simulink model "interpolation_nD_TestGen61"  (R2017b)
settings: Solver=FixedStepDiscrete  StartTime=0.0  StopTime=10.0  RelTol=1e-3
settings Model: Creator=ktrinh  LastModifiedBy=ktrinh
settings DebuggingCC: ParameterOverflowMsg=none

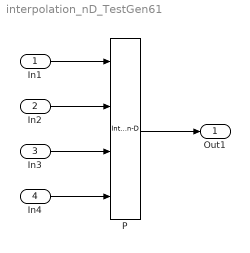
== system interpolation_nD_TestGen61 ==
  In1 : Inport  OutMax=2
  In2 : Inport  Port=2  OutMax=5
  In3 : Inport  Port=3  OutMax=3
  In4 : Inport  Port=4  OutMin=0  OutMax=2
  P : Interpolation_n-D  NumberOfTableDimensions=4  Table=reshape(repmat([4 5 6 7 8;16 19 20 21 22;10 18 23 24 25],2,2),[2,5,3,2])  InterpMethod=Nearest  ValidIndexMayReachLast=on  NumSelectionDims=4  InternalRulePriority=Speed  RndMeth=Simplest  SaturateOnIntegerOverflow=on  IntermediateResultsDataTypeStr=uint16
  Out1 : Outport
  wires:
  In1/1 -> P/1
  In2/1 -> P/2
  In3/1 -> P/3
  In4/1 -> P/4
  P/1 -> Out1/1
